simulink model "bbcSimPIDv2"  (R2024a)
settings: Solver=FixedStepDiscrete  StartTime=0.0  StopTime=0.3  FixedStep=5e-6  RelTol=1e-3
model workspace (MAT data in the model file):
  vIn = 48
libraries: spsSeriesRLCBranchLib x6, spsVoltageMeasurementLib x3, spsDiodeLib x2, spsMosfetLib x2, spsDCVoltageSourceLib x2, spspowerguiLib x2, spsPWMGeneratorDCDCLib x1
settings Model: Creator=mattf  LastModifiedBy=ariellevy

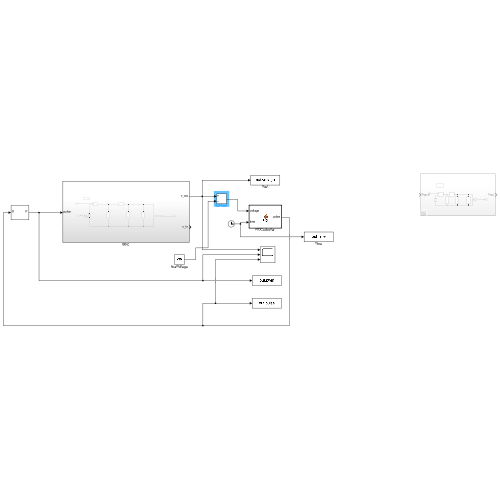
[thumbnail: Simulink's stored preview of the top-level diagram]
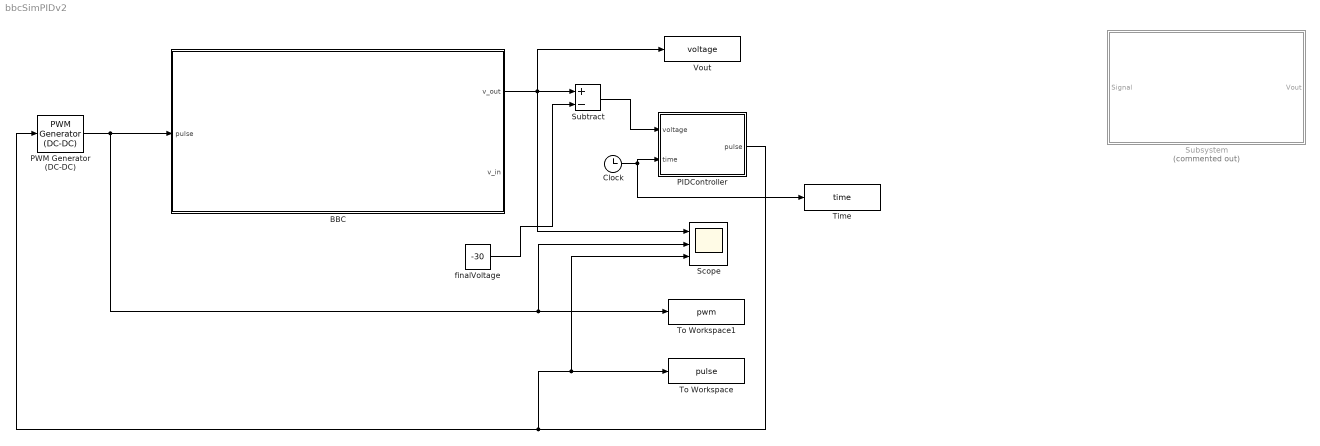
== system bbcSimPIDv2 ==
  BBC : Subsystem
  Clock : Clock
  PIDController : MATLAB Function  TreatAsAtomicUnit=on
  PWM Generator (DC-DC) : spsPWMGeneratorDCDCLib/PWM Generator (DC-DC)  Fsw=7.8e3  Ts=5e-6
  Scope : Scope  NumInputPorts=3
  Subsystem : Subsystem  Commented=on
  Subtract : Sum  Inputs=+-
  Time : ToWorkspace  VariableName=time  SampleTime=-1
  To Workspace : ToWorkspace  VariableName=pulse  SampleTime=-1
  To Workspace1 : ToWorkspace  VariableName=pwm  SampleTime=-1
  Vout : ToWorkspace  VariableName=voltage  SampleTime=-1
  finalVoltage : Constant  Value=-30
  wires:
  Clock/1 -> Time/1, PIDController/2(time)
  BBC/1(v_out) -> Subtract/1, Scope/1, Vout/1
  PWM Generator (DC-DC)/1 -> Scope/2, To Workspace1/1, BBC/1(pulse)
  PIDController/1(pulse) -> PWM Generator (DC-DC)/1, Scope/3, To Workspace/1
  finalVoltage/1 -> Subtract/2
  Subtract/1 -> PIDController/1(voltage)

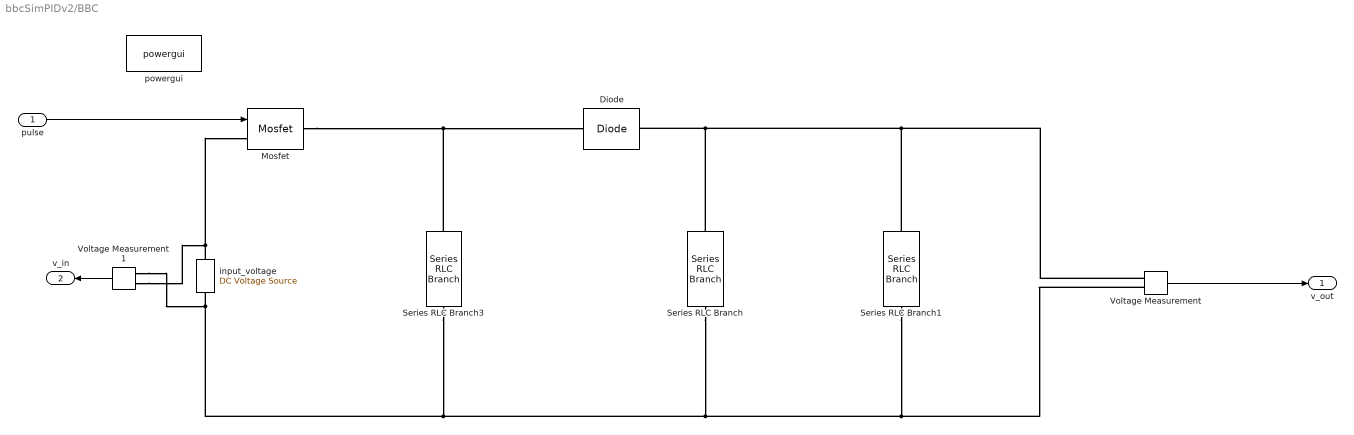
== system bbcSimPIDv2/BBC ==
  pulse : Inport
  Diode : spsDiodeLib/Diode  Ron=0.001  Lon=0  Vf=0.8  IC=0  UseSnubber=0  Rs=500  Cs=250e-9  Measurements=off
  Mosfet : spsMosfetLib/Mosfet  Ron=0.1  Lon=0  Rd=0.01  Vfd=0  IC=0  Rs=1e5  Cs=inf  Measurements=off
  Series RLC Branch : spsSeriesRLCBranchLib/Series RLC Branch  LConnTagsString=__new0  RConnTagsString=__new0  BranchType=C  Resistance=1  Inductance=1e-3  SetiL0=off  InitialCurrent=0  Capacitance=8200e-6  Setx0=off  InitialVoltage=0  Measurements=None
  Series RLC Branch1 : spsSeriesRLCBranchLib/Series RLC Branch  LConnTagsString=__new0  RConnTagsString=__new0  BranchType=R  Resistance=5.1  Inductance=1e-3  SetiL0=off  InitialCurrent=0  Capacitance=1e-6  Setx0=off  InitialVoltage=0  Measurements=None
  Series RLC Branch3 : spsSeriesRLCBranchLib/Series RLC Branch  LConnTagsString=__new0  RConnTagsString=__new0  BranchType=L  Resistance=1  Inductance=220e-6  SetiL0=off  InitialCurrent=0  Capacitance=1e-6  Setx0=off  InitialVoltage=0  Measurements=None
  Voltage Measurement : spsVoltageMeasurementLib/Voltage Measurement  PhasorSimulation=off  OutputType=Complex  PSBequivalent=0
  Voltage Measurement1 : spsVoltageMeasurementLib/Voltage Measurement  PhasorSimulation=off  OutputType=Complex  PSBequivalent=0
  input_voltage : spsDCVoltageSourceLib/DC Voltage Source  Amplitude=48  Measurements=Voltage
  powergui : spspowerguiLib/powergui  Priority=1  SimulationMode=Discrete  SampleTime=5e-6  frequency=60  Iterations=50  frequencyindice=0  Pbase=100e6  ErrMax=1e-4  UnitsV=kV  UnitsW=MW  buscounter=0  FunctionMessages=off  echomessages=off  EnableUseOfTLC=off  CurrentSourceSwitches=off  DisableSnubberDevices=off  DisableRonSwitches=off  DisableVfSwitches=off  DisplayEquations=off  AutomaticDiscreteSolvers=off  SolverType=Tustin/Backward Euler (TBE)  Interpol=off  ExternalGateDelay=off  methode=off  Ts=100  x0status=blocks  SPID=on  SwTol=0  HookPort=off  NonlinearTolerance=1e-4  nMaxIteration=100  ContinueOnMaxIteration=off  RestoreLinks=warning  ResistiveCurrentMeasurement=off  Frange=[0:2:500]  Ylog=off  Xlog=on  ShowGrid=off  save=off  variable=ZData  structure=0  ZoomFFT=off  StartTime=0.0  cycles=1  DisplayStyle=1  fundamental=60  FreqAxis=off  MaxFrequency=1000  frequencyindicesteady=1  RmsSteady=1  display=off
  v_out : Outport
  v_in : Outport  Port=2
  wires:
  pulse/1 -> Mosfet/1
  Voltage Measurement/1 -> v_out/1
  Voltage Measurement1/1 -> v_in/1
  connections:
  input_voltage/RConn1 -- Voltage Measurement1/LConn1 -- Mosfet/LConn1
  Mosfet/RConn1 -- Series RLC Branch3/LConn1 -- Diode/RConn1
  Voltage Measurement/LConn2 -- Series RLC Branch1/RConn1 -- Series RLC Branch/RConn1 -- Series RLC Branch3/RConn1 -- Voltage Measurement1/LConn2 -- input_voltage/LConn1
  Voltage Measurement/LConn1 -- Series RLC Branch1/LConn1 -- Series RLC Branch/LConn1 -- Diode/LConn1

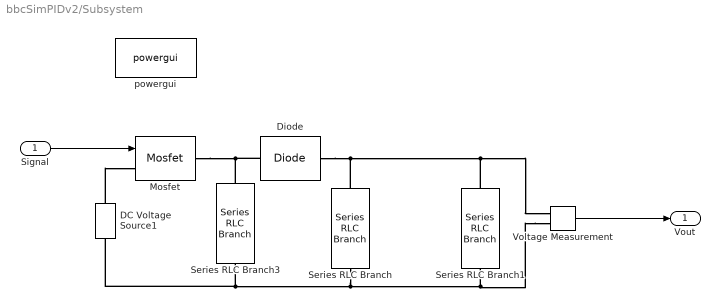
== system bbcSimPIDv2/Subsystem ==
  Signal : Inport
  DC Voltage Source1 : spsDCVoltageSourceLib/DC Voltage Source  Amplitude=100  Measurements=None
  Diode : spsDiodeLib/Diode  Ron=0.001  Lon=0  Vf=0.8  IC=0  UseSnubber=0  Rs=500  Cs=250e-9  Measurements=off
  Mosfet : spsMosfetLib/Mosfet  Ron=0.1  Lon=0  Rd=0.01  Vfd=0  IC=0  Rs=1e5  Cs=inf  Measurements=off
  Series RLC Branch : spsSeriesRLCBranchLib/Series RLC Branch  LConnTagsString=__new0  RConnTagsString=__new0  BranchType=C  Resistance=1  Inductance=1e-3  SetiL0=off  InitialCurrent=0  Capacitance=1e-6  Setx0=off  InitialVoltage=0  Measurements=None
  Series RLC Branch1 : spsSeriesRLCBranchLib/Series RLC Branch  LConnTagsString=__new0  RConnTagsString=__new0  BranchType=R  Resistance=1  Inductance=1e-3  SetiL0=off  InitialCurrent=0  Capacitance=1e-6  Setx0=off  InitialVoltage=0  Measurements=None
  Series RLC Branch3 : spsSeriesRLCBranchLib/Series RLC Branch  LConnTagsString=__new0  RConnTagsString=__new0  BranchType=L  Resistance=1  Inductance=1e-3  SetiL0=off  InitialCurrent=0  Capacitance=1e-6  Setx0=off  InitialVoltage=0  Measurements=None
  Voltage Measurement : spsVoltageMeasurementLib/Voltage Measurement  PhasorSimulation=off  OutputType=Complex  PSBequivalent=0
  powergui : spspowerguiLib/powergui  Priority=1  SimulationMode=Discrete  SampleTime=0.001  frequency=60  Iterations=50  frequencyindice=0  Pbase=100e6  ErrMax=1e-4  UnitsV=kV  UnitsW=MW  buscounter=0  FunctionMessages=off  echomessages=off  EnableUseOfTLC=off  CurrentSourceSwitches=off  DisableSnubberDevices=off  DisableRonSwitches=off  DisableVfSwitches=off  DisplayEquations=off  AutomaticDiscreteSolvers=off  SolverType=Tustin/Backward Euler (TBE)  Interpol=off  ExternalGateDelay=off  methode=off  Ts=100  x0status=blocks  SPID=on  SwTol=0  HookPort=off  NonlinearTolerance=1e-4  nMaxIteration=100  ContinueOnMaxIteration=off  RestoreLinks=warning  ResistiveCurrentMeasurement=off  Frange=[0:2:500]  Ylog=off  Xlog=on  ShowGrid=off  save=off  variable=ZData  structure=0  ZoomFFT=off  StartTime=0.0  cycles=1  DisplayStyle=1  fundamental=60  FreqAxis=off  MaxFrequency=1000  frequencyindicesteady=1  RmsSteady=1  display=off
  Vout : Outport
  wires:
  Voltage Measurement/1 -> Vout/1
  Signal/1 -> Mosfet/1
  connections:
  Diode/LConn1 -- Series RLC Branch/LConn1 -- Series RLC Branch1/LConn1 -- Voltage Measurement/LConn1
  Voltage Measurement/LConn2 -- Series RLC Branch/RConn1 -- Series RLC Branch3/RConn1 -- DC Voltage Source1/LConn1 -- Series RLC Branch1/RConn1
  Diode/RConn1 -- Series RLC Branch3/LConn1 -- Mosfet/RConn1
  DC Voltage Source1/RConn1 -- Mosfet/LConn1

== matlab function bbcSimPIDv2/PIDController ==
  settings: updateMethod=DISCRETE
  data: voltage input; pulse output; time input
function pulse = PID(voltage, time)

    % call extrinsic python function
    coder.extrinsic('py.PIDControllerBBC.controller_call');

    % Call Python function and return result
    pulse = coder.nullcopy(zeros(1,1)); % no clue why, but this is need.
    pulse = double(py.PIDControllerBBC.controller_call(voltage, time));
    end
